simulink model "Part33DofSim"  (R2019a)
settings: Solver=VariableStepAuto  StartTime=0.0  StopTime=10  RelTol=1e-3
values from neighbouring files (symbols this model uses):
  A = [-c/ms c/ms;c/mu -c/mu]    [Part12b.m]    (also in Part33DofPar.m = [a11 a12 a13 a14; Part3BicyclePar.m = [-(caf+car)/(u*M) -((a*caf-b*car)/(u*M)+u); part23.m = [a11 a12 a13)
  a = 1.2    [Part33DofPar.m]    (also in Part3BicyclePar.m; part23.m)
  B = [-ks/ms ks/ms;ks/mu -ks/mu-kt/mu]    [Part12b.m]    (also in Part33DofPar.m = [b1;b2;b3;b4]; Part3BicyclePar.m = [caf/M;a*caf/Iz]; part23.m = [b1;b2;b4])
  b = 1.4    [Part33DofPar.m]    (also in Part3BicyclePar.m; part23.m)
  delta = 2.5/180*pi    (= 0.0436332312999)    [Part33DofPar.m]    (also in Part3BicyclePar.m)
  ksbrf = 0.1    [Part33DofPar.m]    (also in Part3BicyclePar.m; part23.m)
  ksbrr = 0.1    [Part33DofPar.m]    (also in Part3BicyclePar.m; part23.m)
libraries: simulink x1

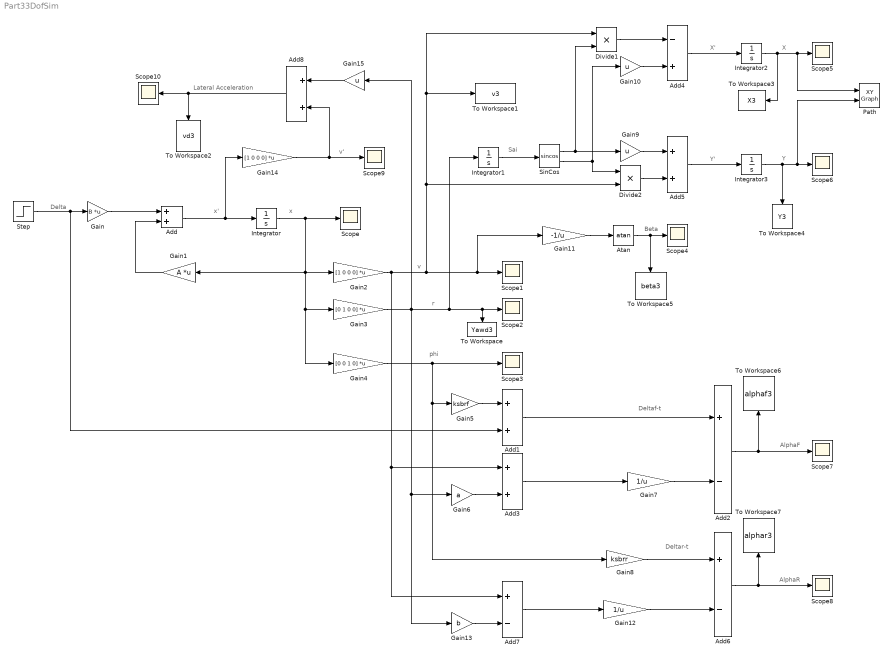
== system Part33DofSim ==
  note: Lateral Acceleration
  note: v'
  note: Deltaf-t
  note: phi
  note: r
  note: v
  note: Delta
  note: x
  note: x'
  note: Beta
  note: X'
  note: X
  note: Y
  note: Y'
  note: Sai
  note: AlphaF
  note: Deltar-t
  note: AlphaR
  Add{,1,3,5,8} (5 alike) : Sum
  Add2 : Sum  Inputs=+-
  Add4 : Sum  Inputs=-+
  Add6 : Sum  Inputs=+-
  Add7 : Sum  Inputs=+-
  Atan : Trigonometry  Operator=atan
  Divide1 : Product  Inputs=**
  Divide2 : Product  Inputs=**
  Gain : Gain  Gain=B  Multiplication=Matrix(K*u)
  Gain1 : Gain  Gain=A  Multiplication=Matrix(K*u)
  Gain10 : Gain  Gain=u
  Gain11 : Gain  Gain=-1/u
  Gain12 : Gain  Gain=1/u
  Gain13 : Gain  Gain=b
  Gain14 : Gain  Gain=[1 0 0 0]  Multiplication=Matrix(K*u)
  Gain15 : Gain  Gain=u
  Gain2 : Gain  Gain=[1 0 0 0]  Multiplication=Matrix(K*u)
  Gain3 : Gain  Gain=[0 1 0 0]  Multiplication=Matrix(K*u)
  Gain4 : Gain  Gain=[0 0 1 0]  Multiplication=Matrix(K*u)
  Gain5 : Gain  Gain=ksbrf
  Gain6 : Gain  Gain=a
  Gain7 : Gain  Gain=1/u
  Gain8 : Gain  Gain=ksbrr
  Gain9 : Gain  Gain=u
  Integrator{,1..3} (4 alike) : Integrator
  Path : simulink/Sinks/XY Graph  xmin=-200  xmax=300  ymin=-200  ymax=300  st=-1
  Scope{,1..10} (11 alike) : Scope
  SinCos : Trigonometry  Operator=sincos
  Step : Step  After=delta  SampleTime=0
  To Workspace : ToWorkspace  VariableName=Yawd3  SaveFormat=Timeseries  SampleTime=-1
  To Workspace1 : ToWorkspace  VariableName=v3  SaveFormat=Timeseries  SampleTime=-1
  To Workspace2 : ToWorkspace  VariableName=vd3  SaveFormat=Timeseries  SampleTime=-1
  To Workspace3 : ToWorkspace  VariableName=X3  SaveFormat=Timeseries  SampleTime=-1
  To Workspace4 : ToWorkspace  VariableName=Y3  SaveFormat=Timeseries  SampleTime=-1
  To Workspace5 : ToWorkspace  VariableName=beta3  SaveFormat=Timeseries  SampleTime=-1
  To Workspace6 : ToWorkspace  VariableName=alphaf3  SaveFormat=Timeseries  SampleTime=-1
  To Workspace7 : ToWorkspace  VariableName=alphar3  SaveFormat=Timeseries  SampleTime=-1
  wires:
  Step/1 -> Add1/2, Gain/1
  Gain/1 -> Add/1
  Add/1 -> Gain14/1, Integrator/1
  Integrator/1 -> Gain4/1, Gain3/1, Gain2/1, Gain1/1, Scope/1
  Gain1/1 -> Add/2
  Gain4/1 -> Gain8/1, Gain5/1, Scope3/1
  Gain11/1 -> Atan/1
  Atan/1 -> To Workspace5/1, Scope4/1
  SinCos/1 -> Gain9/1, Divide1/2
  Gain3/1 -> Gain13/1, Gain6/1, Gain15/1, Integrator1/1, To Workspace/1, Scope2/1
  Integrator2/1 -> To Workspace3/1, Path/1, Scope5/1
  Divide1/1 -> Add4/1
  Integrator3/1 -> To Workspace4/1, Path/2, Scope6/1
  Add5/1 -> Integrator3/1
  Add4/1 -> Integrator2/1
  Gain2/1 -> Add7/1, Add3/1, Divide2/2, Divide1/1, To Workspace1/1, Gain11/1, Scope1/1
  SinCos/2 -> Divide2/1, Gain10/1
  Gain10/1 -> Add4/2
  Integrator1/1 -> SinCos/1
  Divide2/1 -> Add5/2
  Gain9/1 -> Add5/1
  Gain5/1 -> Add1/1
  Add1/1 -> Add2/1
  Gain6/1 -> Add3/2
  Add3/1 -> Gain7/1
  Gain7/1 -> Add2/2
  Add2/1 -> To Workspace6/1, Scope7/1
  Gain8/1 -> Add6/1
  Add7/1 -> Gain12/1
  Gain12/1 -> Add6/2
  Gain13/1 -> Add7/2
  Add6/1 -> To Workspace7/1, Scope8/1
  Gain14/1 -> Add8/2, Scope9/1
  Gain15/1 -> Add8/1
  Add8/1 -> Scope10/1, To Workspace2/1
